simulink model "simulink_model"  (R2021b)
settings: Solver=VariableStepAuto  StartTime=0.0  StopTime=16384  RelTol=1e-3
model workspace (MAT data in the model file):
  deg = 4
undefined symbols (not defined in the file or in its folder): DiscIntNeverNeededParam
libraries: ctrlSharedLib x2
settings Model: Creator=Enes  LastModifiedBy=Enes
settings DataIOCC: ExternalInput=signal_1  OutputSaveName=Simulation_Output

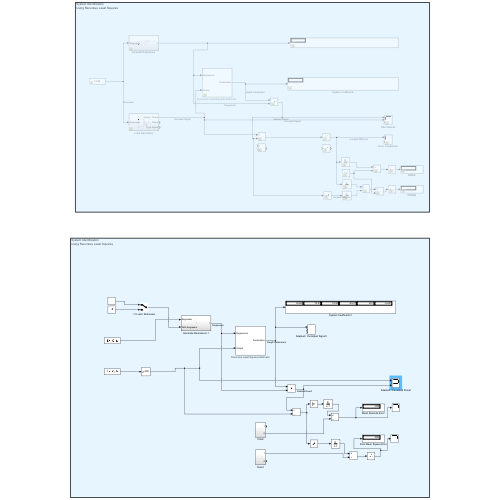
[thumbnail: Simulink's stored preview of the top-level diagram]
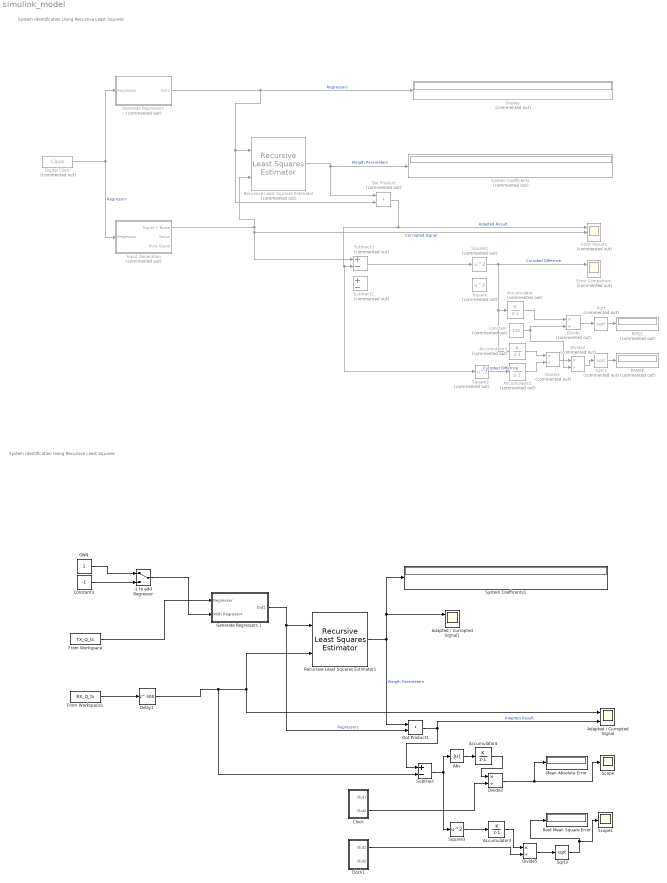
== system simulink_model ==
  note: System Identification
      | Using Recursive Least Squares
  note: System Identification
      | Using Recursive Least Squares
  -1 to add  Regressor : ManualSwitch
  Abs : Abs
  Accumulator : DiscreteIntegrator  Commented=on  IntegratorMethod=Accumulation: Forward Euler  SampleTime=-1  ICPrevOutput=DiscIntNeverNeededParam  ICPrevScaledInput=DiscIntNeverNeededParam
  Accumulator1 : DiscreteIntegrator  Commented=on  IntegratorMethod=Accumulation: Forward Euler  SampleTime=-1  ICPrevOutput=DiscIntNeverNeededParam  ICPrevScaledInput=DiscIntNeverNeededParam
  Accumulator2 : DiscreteIntegrator  Commented=on  IntegratorMethod=Accumulation: Forward Euler  SampleTime=-1  ICPrevOutput=DiscIntNeverNeededParam  ICPrevScaledInput=DiscIntNeverNeededParam
  Accumulator3 : DiscreteIntegrator  IntegratorMethod=Accumulation: Forward Euler  SampleTime=-1  ICPrevOutput=DiscIntNeverNeededParam  ICPrevScaledInput=DiscIntNeverNeededParam
  Accumulator4 : DiscreteIntegrator  IntegratorMethod=Accumulation: Forward Euler  SampleTime=-1  ICPrevOutput=DiscIntNeverNeededParam  ICPrevScaledInput=DiscIntNeverNeededParam
  Adapted / Curropted Signal : Scope  NumInputPorts=3
  Adapted / Curropted Signal1 : Scope  NumInputPorts=3
  Clock : Subsystem
  Clock1 : Subsystem
  Constant : Constant  Commented=on  Value=150
  Constant3 : Constant  Value=-1
  Delay1 : Delay  DelayLength=300
  Digital Clock : DigitalClock  Commented=on
  Display : Display  Commented=on
  Divide : Product  Commented=on  Inputs=*/
  Divide1 : Product  Commented=on  Inputs=*/
  Divide2 : Product  Commented=on  Inputs=*/
  Divide3 : Product  Inputs=*/
  Divide5 : Product  Inputs=*/
  Dot Product : DotProduct  Commented=on  InputSameDT=on  OutDataTypeStr=Inherit: Inherit via internal rule
  Dot Product1 : DotProduct  InputSameDT=on  OutDataTypeStr=Inherit: Inherit via internal rule
  Error Comperison : Scope  Commented=on  NumInputPorts=2
  Filter Results : Scope  Commented=on  NumInputPorts=3
  From Workspace : FromWorkspace  VariableName=TX_Q_ts  SampleTime=-1
  From Workspace1 : FromWorkspace  VariableName=RX_Q_ts  SampleTime=-1
  "Generate Regressors " : Subsystem  Commented=on
  Generate Regressors 1 : Subsystem
  Input Generation : Subsystem  Commented=on
  Mean Absolute Error : Display
  ONN : Constant
  PRMSE : Display  Commented=on
  RMSE : Display  Commented=on
  Recursive Least Squares Estimator : ctrlSharedLib/Recursive Least Squares Estimator  Tag=Recursive Least Squares Estimator  Description=Recursive Least Squares Estimator  Commented=on  InitialEstimateSource=None  InitialParameterData=10  P0=1e4  InitialRegressors=0  InitialOutputs=0  History=Infinite  WindowLength=3  EstimationMethod=Forgetting Factor  AdaptationParameter=0.95  HasTimeVaryingAdaptationParameter=off  NormalizationBias=eps  OutputError=off  OutputP=off  AddEnablePort=off  InputProcessing=Sample-based  Ts=-1
      settings: AttributesFormatString=Recursive Least Squares Estimator  SourceProductBaseCode=CT,ID
  Recursive Least Squares Estimator1 : ctrlSharedLib/Recursive Least Squares Estimator  Tag=Recursive Least Squares Estimator  Description=Recursive Least Squares Estimator  InitialEstimateSource=None  InitialParameterData=6  P0=1e4  InitialRegressors=0  InitialOutputs=0  History=Infinite  WindowLength=3  EstimationMethod=Forgetting Factor  AdaptationParameter=0.95  HasTimeVaryingAdaptationParameter=off  NormalizationBias=eps  OutputError=off  OutputP=off  AddEnablePort=off  InputProcessing=Sample-based  Ts=-1
      settings: AttributesFormatString=Recursive Least Squares Estimator  SourceProductBaseCode=CT,ID
  Root Mean Square Error : Display
  Scope : Scope
  Scope1 : Scope
  Sqrt : Sqrt  Commented=on  SaturateOnIntegerOverflow=on
  Sqrt1 : Sqrt  Commented=on  SaturateOnIntegerOverflow=on
  Sqrt3 : Sqrt  SaturateOnIntegerOverflow=on
  Square : Math  Commented=on  Operator=square  SaturateOnIntegerOverflow=on
  Square1 : Math  Commented=on  Operator=square  SaturateOnIntegerOverflow=on
  Square2 : Math  Commented=on  Operator=square  SaturateOnIntegerOverflow=on
  Square3 : Math  Operator=square  SaturateOnIntegerOverflow=on
  Subtract : Sum  Inputs=+-
  Subtract2 : Sum  Commented=on  Inputs=+-
  Subtract3 : Sum  Commented=on  Inputs=+-
  System Coefficents : Display  Commented=on
  System Coefficents1 : Display
  wires:
  Digital Clock/1 -> "Generate Regressors "/1(Regressor), Input Generation/1(Regressor)  "Regressor"
  Recursive Least Squares Estimator/1 -> System Coefficents/1, Dot Product/1  "Weigth Parameters"
  Dot Product/1 -> Square2/1, Subtract3/2, Filter Results/1  "Adapted Result"
  Subtract3/1 -> Square1/1
  Square1/1 -> Accumulator1/1, Accumulator/1, Error Comperison/1  "Currpted Differnce"
  "Generate Regressors "/1(Out1) -> Display/1, Dot Product/2, Recursive Least Squares Estimator/1  "Regressors"
  Input Generation/1(Signal + Noise) -> Filter Results/2, Subtract3/1, Recursive Least Squares Estimator/2  "Corropted Signal"
  Accumulator/1 -> Divide/1
  Constant/1 -> Divide2/2, Divide/2
  Divide/1 -> Sqrt/1
  Sqrt/1 -> RMSE/1
  Accumulator2/1 -> Divide1/2
  Accumulator1/1 -> Divide1/1
  Square2/1 -> Accumulator2/1  "Currpted Differnce"
  Sqrt1/1 -> PRMSE/1
  Divide1/1 -> Divide2/1
  Divide2/1 -> Sqrt1/1
  Generate Regressors 1/1(Out1) -> Dot Product1/2, Recursive Least Squares Estimator1/1  "Regressors"
  Recursive Least Squares Estimator1/1 -> Dot Product1/1, System Coefficents1/1, Adapted / Curropted Signal1/1  "Weigth Parameters"
  Dot Product1/1 -> Adapted / Curropted Signal/3, Subtract/1  "Adapted Result"
  Subtract/1 -> Abs/1, Square3/1
  -1 to add  Regressor/1 -> Generate Regressors 1/2(With Regressor)
  ONN/1 -> -1 to add  Regressor/1
  Constant3/1 -> -1 to add  Regressor/2
  From Workspace1/1 -> Delay1/1
  From Workspace/1 -> Generate Regressors 1/1(Regressor)
  Delay1/1 -> Subtract/2, Adapted / Curropted Signal/1, Recursive Least Squares Estimator1/2
  Clock/2(Out2) -> Divide3/2
  Divide3/1 -> Scope/1, Mean Absolute Error/1
  Clock1/1(Out1) -> Divide5/2
  Square3/1 -> Accumulator3/1
  Accumulator3/1 -> Divide5/1
  Divide5/1 -> Sqrt3/1
  Sqrt3/1 -> Scope1/1, Root Mean Square Error/1
  Abs/1 -> Accumulator4/1
  Accumulator4/1 -> Divide3/1

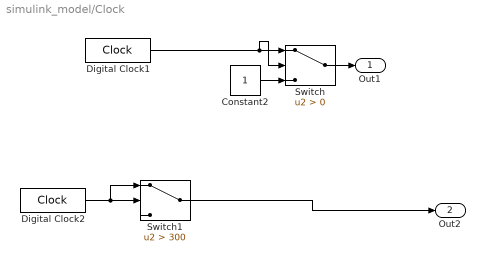
== system simulink_model/Clock ==
  Constant2 : Constant
  Digital Clock1 : DigitalClock
  Digital Clock2 : DigitalClock
  Switch : Switch  Criteria=u2 > Threshold
  Switch1 : Switch  Criteria=u2 > Threshold  Threshold=300
  Out1 : Outport
  Out2 : Outport  Port=2
  wires:
  Digital Clock1/1 -> Switch/1, Switch/2
  Switch/1 -> Out1/1
  Constant2/1 -> Switch/3
  Switch1/1 -> Out2/1
  Digital Clock2/1 -> Switch1/1, Switch1/2

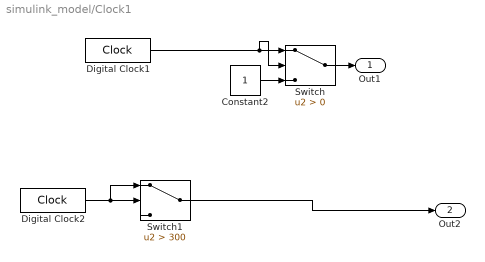
== system simulink_model/Clock1 ==
  Constant2 : Constant
  Digital Clock1 : DigitalClock
  Digital Clock2 : DigitalClock
  Switch : Switch  Criteria=u2 > Threshold
  Switch1 : Switch  Criteria=u2 > Threshold  Threshold=300
  Out1 : Outport
  Out2 : Outport  Port=2
  wires:
  Digital Clock2/1 -> Switch1/2, Switch1/1
  Switch1/1 -> Out2/1
  Constant2/1 -> Switch/3
  Switch/1 -> Out1/1
  Digital Clock1/1 -> Switch/2, Switch/1

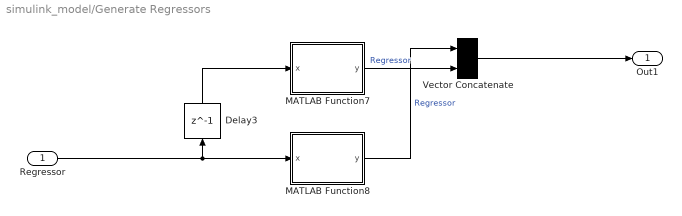
== system simulink_model/Generate Regressors  ==
  Regressor : Inport
  Delay3 : Delay  DelayLength=1  SampleTime=1
  MATLAB Function7 : MATLAB Function  TreatAsAtomicUnit=on
  MATLAB Function8 : MATLAB Function  TreatAsAtomicUnit=on
  Vector Concatenate : Concatenate
  Out1 : Outport
  wires:
  MATLAB Function7/1(y) -> Vector Concatenate/2  "Regressor"
  Vector Concatenate/1 -> Out1/1
  MATLAB Function8/1(y) -> Vector Concatenate/1  "Regressor"
  Delay3/1 -> MATLAB Function7/1(x)
  Regressor/1 -> MATLAB Function8/1(x), Delay3/1

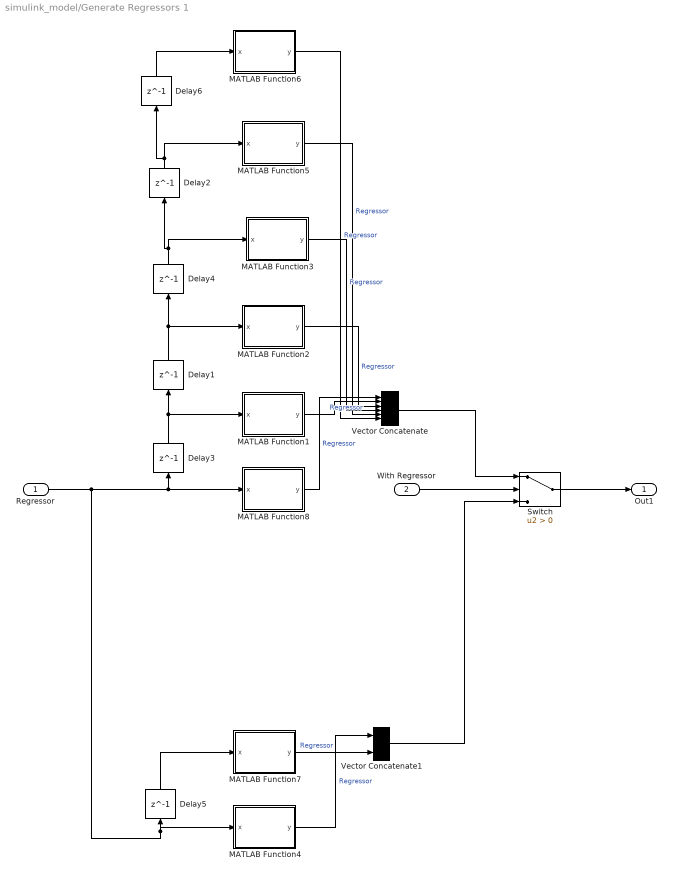
== system simulink_model/Generate Regressors 1 ==
  Regressor : Inport
  With Regressor : Inport  Port=2
  Delay{1..6} (6 alike) : Delay  DelayLength=1  SampleTime=1
  MATLAB Function1 : MATLAB Function  TreatAsAtomicUnit=on
  MATLAB Function2 : MATLAB Function  TreatAsAtomicUnit=on
  MATLAB Function3 : MATLAB Function  TreatAsAtomicUnit=on
  MATLAB Function4 : MATLAB Function  TreatAsAtomicUnit=on
  MATLAB Function5 : MATLAB Function  TreatAsAtomicUnit=on
  MATLAB Function6 : MATLAB Function  TreatAsAtomicUnit=on
  MATLAB Function7 : MATLAB Function  TreatAsAtomicUnit=on
  MATLAB Function8 : MATLAB Function  TreatAsAtomicUnit=on
  Switch : Switch  Criteria=u2 > Threshold
  Vector Concatenate : Concatenate  NumInputs=6
  Vector Concatenate1 : Concatenate
  Out1 : Outport
  wires:
  MATLAB Function1/1(y) -> Vector Concatenate/2  "Regressor"
  Vector Concatenate/1 -> Switch/1
  MATLAB Function8/1(y) -> Vector Concatenate/1  "Regressor"
  Delay3/1 -> Delay1/1, MATLAB Function1/1(x)
  Regressor/1 -> MATLAB Function4/1(x), Delay5/1, MATLAB Function8/1(x), Delay3/1
  Delay1/1 -> Delay4/1, MATLAB Function2/1(x)
  MATLAB Function2/1(y) -> Vector Concatenate/3  "Regressor"
  Delay4/1 -> Delay2/1, MATLAB Function3/1(x)
  MATLAB Function3/1(y) -> Vector Concatenate/4  "Regressor"
  MATLAB Function7/1(y) -> Vector Concatenate1/2  "Regressor"
  Vector Concatenate1/1 -> Switch/3
  MATLAB Function4/1(y) -> Vector Concatenate1/1  "Regressor"
  Delay5/1 -> MATLAB Function7/1(x)
  With Regressor/1 -> Switch/2
  Switch/1 -> Out1/1
  MATLAB Function5/1(y) -> Vector Concatenate/5  "Regressor"
  Delay2/1 -> Delay6/1, MATLAB Function5/1(x)
  Delay6/1 -> MATLAB Function6/1(x)
  MATLAB Function6/1(y) -> Vector Concatenate/6  "Regressor"

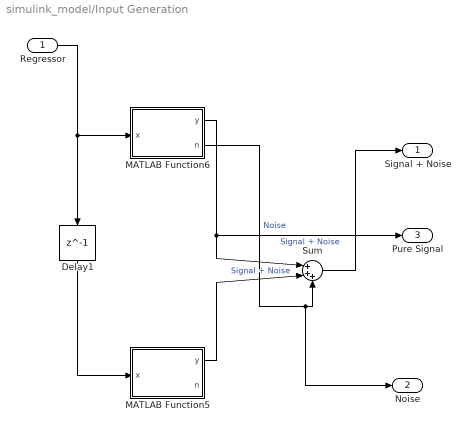
== system simulink_model/Input Generation ==
  Regressor : Inport
  Delay1 : Delay  DelayLength=1  SampleTime=1
  MATLAB Function5 : MATLAB Function  TreatAsAtomicUnit=on
  MATLAB Function6 : MATLAB Function  TreatAsAtomicUnit=on
  Sum : Sum  Inputs=|+++
  Signal + Noise : Outport
  Noise : Outport  Port=2
  Pure Signal : Outport  Port=3
  wires:
  MATLAB Function6/2(n) -> Noise/1, Sum/3  "Noise"
  Delay1/1 -> MATLAB Function5/1(x)
  MATLAB Function5/1(y) -> Sum/2  "Signal + Noise"
  MATLAB Function6/1(y) -> Sum/1, Pure Signal/1  "Signal + Noise"
  Regressor/1 -> Delay1/1, MATLAB Function6/1(x)
  Sum/1 -> Signal + Noise/1

== matlab function simulink_model/Generate Regressors /MATLAB Function8 ==
  data: x input; y output
function y = fcn(x)


c = sin(x*pi/5);

y = [c^4,c^3,c^2,c,1];

== matlab function simulink_model/Generate Regressors 1/MATLAB Function8 ==
  data: x input; y output
function y = fcn(x)

y = x;

== matlab function simulink_model/Generate Regressors 1/MATLAB Function1 ==
  data: x input; y output
function y = fcn(x)

y = x;

== matlab function simulink_model/Generate Regressors 1/MATLAB Function3 ==
  data: x input; y output
function y = fcn(x)

y = x;

== matlab function simulink_model/Input Generation/MATLAB Function5 ==
  data: x input; y output; n output
function [y,n] = fcn(x)


n=10*normrnd(0,2);
c = sin(x*pi/5);

% if mod(x,4) == 3 
%     n=5*normrnd(0,2);
% else
%     n=2*normrnd(0,2);
% end

y = 0.09*c^4 -2.2*c^3 + 8.0*c^2 -14*c;

== matlab function simulink_model/Input Generation/MATLAB Function6 ==
  data: x input; y output; n output
function [y,n] = fcn(x)


n=0.5*normrnd(0,2);
c = sin(x*pi/5);

% if mod(x,4) == 3 
%     n=5*normrnd(0,2);
% else
%     n=2*normrnd(0,2);
% end

y = 0.07*c^4 -1.9*c^3 + 7.9*c^2 -13*c;

== matlab function simulink_model/Generate Regressors /MATLAB Function7 ==
  data: x input; y output
function y = fcn(x)

c = sin(x*pi/5);

y = [c^4,c^3,c^2,c,1];

== matlab function simulink_model/Generate Regressors 1/MATLAB Function5 ==
  data: x input; y output
function y = fcn(x)

y = x;

== matlab function simulink_model/Generate Regressors 1/MATLAB Function6 ==
  data: x input; y output
function y = fcn(x)

y = x;

== matlab function simulink_model/Generate Regressors 1/MATLAB Function2 ==
  data: x input; y output
function y = fcn(x)

y = x;

== matlab function simulink_model/Generate Regressors 1/MATLAB Function4 ==
  data: x input; y output
function y = fcn(x)

c=x;

y = [c^2,c,1];

== matlab function simulink_model/Generate Regressors 1/MATLAB Function7 ==
  data: x input; y output
function y = fcn(x)

c = x;

y = [c^2,c,1];
